simulink model "Model_tmp"  (Simulink 8.5)
settings: Solver=ode3  StartTime=0.0  StopTime=10.0  RelTol=1e-3
PreLoadFcn:
  | % Bus object: subBus
  | clear elems;
  | elems(1) = Simulink.BusElement;
  | elems(1).Name = 'chirp';
  | elems(1).Dimensions = 2;
  | elems(1).DimensionsMode = 'Fixed';
  | elems(1).DataType = 'double';
  | elems(1).SampleTime = -1;
  | elems(1).Complexity = 'real';
  | elems(1).Min = [];
  | elems(1).Max = [];
  | elems(1).DocUnits = '';
  | elems(1).Description = '';
  | 
  | elems(2) = Simulink.BusElement;
  | elems(2).Name = 'sine';
  | elems(2).Dimensions = 3;
  | elems(2).DimensionsMode = 'Fixed';
  | elems(2).DataType = 'int32';
  | elems(2).SampleTime = -1;
  | elems(2).Complexity = 'real';
  | elems(2).Min = [];
  | elems(2).Max = [];
  | elems(2).DocUnits = '';
  | elems(2).Description = '';
  | 
  | subBus2 = Simulink.Bus;
  | subBus2.HeaderFile = '';
  | subBus2.Description = '';
  | subBus2.DataScope = 'Auto';
  | subBus2.Alignment = -1;
  | subBus2.Elements = elems;
  | clear elems;
  | assignin('base','subBus2', subBus2);
settings Model: Creator=arnaud  LastModifiedBy=ktrinh  CovSFcnEnable=off
settings DataIOCC: SaveFormat=Structure  SignalLoggingSaveFormat=Dataset  SaveOutput=off  SaveTime=off
settings OptimizationCC: ExpressionDepthLimit=128
settings DebuggingCC: UnderspecifiedInitializationDetection=Simplified  MergeDetectMultiDrivingBlocksExec=error  SolverPrmCheckMsg=warning  FcnCallInpInsideContextMsg=EnableAllAsWarning  BusObjectLabelMismatch=error  ModelReferenceDataLoggingMessage=none  StateNameClashWarn=none
settings ModelReferenceCC: ModelReferenceNumInstancesAllowed=Single
settings GRTTargetCC: CombineOutputUpdateFcns=on  GRTInterface=off

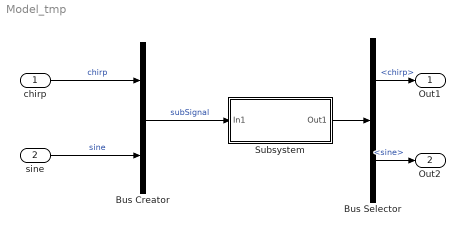
== system Model_tmp ==
  chirp : Inport
  sine : Inport  Port=2
  Bus Selector : BusSelector  OutputSignals=chirp,sine
  Bus Creator : BusCreator  Inputs=2  OutDataTypeStr=Bus: subBus  NonVirtualBus=on
      settings: AttributesFormatString=SubBus  InheritFromInputs=off
  Subsystem : Subsystem  TreatAsAtomicUnit=on
  Out1 : Outport  SampleTime=0
  Out2 : Outport  Port=2  SampleTime=0
  wires:
  Bus Creator/1 -> Subsystem/1(In1)  "subSignal"
  chirp/1 -> Bus Creator/1  "chirp"
  sine/1 -> Bus Creator/2  "sine"
  Subsystem/1(Out1) -> Bus Selector/1
  Bus Selector/1 -> Out1/1  "<chirp>"
  Bus Selector/2 -> Out2/1  "<sine>"

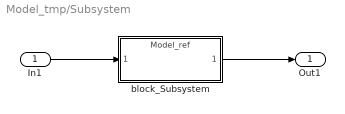
== system Model_tmp/Subsystem ==
  In1 : Inport  OutDataTypeStr=Bus: subBus
  block_Subsystem : ModelReference  ModelNameDialog=Model_ref.mdl  SimulationMode=Normal  ModelReferenceVersion=1.19
  Out1 : Outport  OutDataTypeStr=Bus: subBus2
  wires:
  In1/1 -> block_Subsystem/1
  block_Subsystem/1 -> Out1/1
